simulink model "mrac_model"  (R2022a)
settings: Solver=VariableStepAuto  StartTime=0.0  StopTime=100  RelTol=1e-3
values from neighbouring files (symbols this model uses):
  params = getParamsMRAC(0.5, 1, 10e-8, 0.1, 1)    [mrac.m]
libraries: slctrlblks x1
settings Model: Creator=mateusz  LastModifiedBy=mateusz

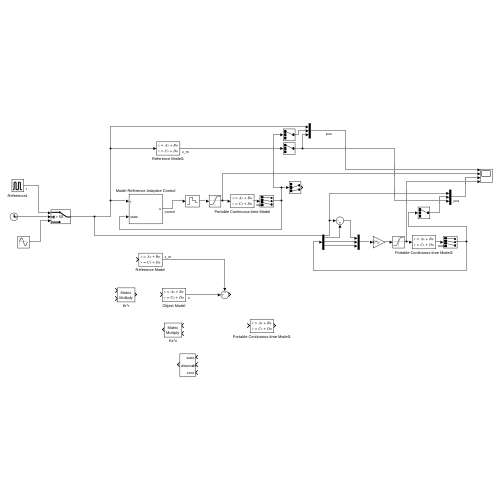
[thumbnail: Simulink's stored preview of the top-level diagram]
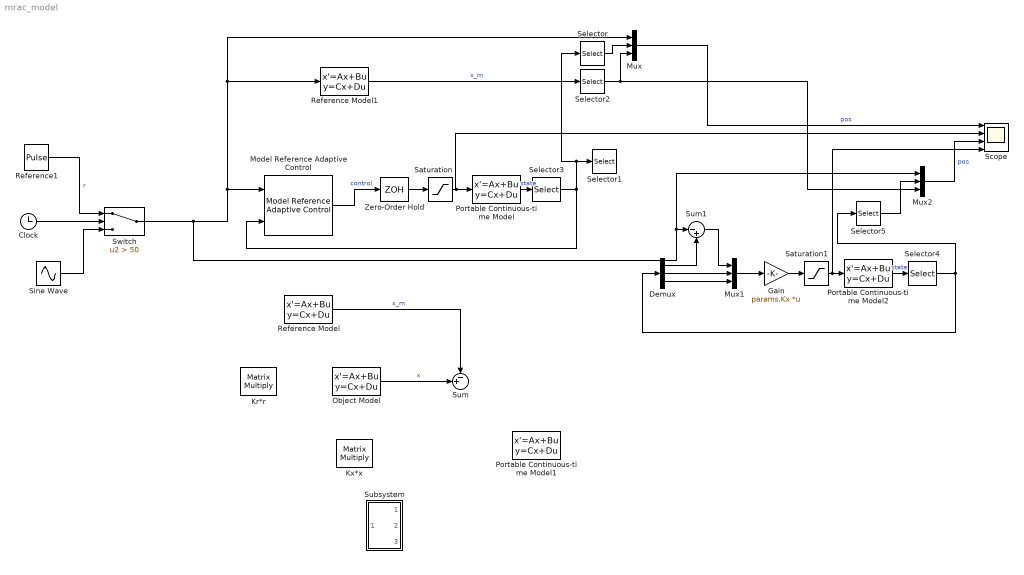
== system mrac_model ==
  Clock : Clock
  Demux : Demux  Outputs=3
  Gain : Gain  Gain=params.Kx  Multiplication=Matrix(K*u)
  Kr*r : Product  Multiplication=Matrix(*)
  Kx*x : Product  Multiplication=Matrix(*)
  Model Reference Adaptive Control : slctrlblks/Model Reference Adaptive Control  selectType=Direct  A=params.A  B=params.B  Ahat=0  ALrEnable=on  gamma_a=1  ALrEnableMod=on  Bhat=1  BLrEnable=on  gamma_b=1  BLrEnableMod=on  externalKtauEnable=off  k_tau=-1  estParamOutput=off  Am=params.A + params.B*params.Kx  Bm=params.B*params.Kr  kx=params.Kx  FBLrEnable=on  gamma_kx=params.gamma_x  FBLrEnableMod=on  kr=params.Kr  FFLrEnable=off  gamma_kr=params.gamma_x  FFLrEnableMod=off  AdaptEnable=on  gamma=params.gamma_w  WLrEnableMod=on  Q=params.Q(1,1)  FeatureTypeOptions=Radial Basis Function  nCen=4  cSpanMin=-1  cSpanMax=1  cSig=5  adaptiveCntrlOutport=off  modChoice=None  sigma_val=0.1
      settings: SourceProductBaseCode=SD
  Mux : Mux  Inputs=3
  Mux1 : Mux  Inputs=3
  Mux2 : Mux  Inputs=3
  Object Model : StateSpace  A=|  B=[0;0;0;2.59e4];  C=eye(4,4)  D=zeros(4,1)  InitialCondition=0
      | [0  1  0    0;
      |      0 -5  4.5  0;
      |      0  0 -0.7108*2  2*23.6012;
      |      0  0 -5.3898 -4040];
  Portable Continuous-time Model : StateSpace  A=|  B=[0;0;0;2.59e4];  C=eye(4,4)  D=zeros(4,1)  InitialCondition=0
      | [0  1  0    0;
      |      0 -5  4.5  0;
      |      0  0 -0.7108*2  2*23.6012;
      |      0  0 -5.3898 -4040];
  Portable Continuous-time Model1 : StateSpace  A=|  B=[0;0;0;2.59e4];  C=eye(4,4)  D=zeros(4,1)  InitialCondition=0
      | [0  1  0    0;
      |      0 -5  4.5  0;
      |      0  0 -0.7108*2  2*23.6012;
      |      0  0 -5.3898 -4040];
  Portable Continuous-time Model2 : StateSpace  A=|  B=[0;0;0;2.59e4];  C=eye(4,4)  D=zeros(4,1)  InitialCondition=0
      | [0  1  0    0;
      |      0 -5  4.5  0;
      |      0  0 -0.7108*2  2*23.6012;
      |      0  0 -5.3898 -4040];
  Reference Model : StateSpace  InitialCondition=0
  Reference Model1 : StateSpace  A=params.Am  B=params.Bm  C=eye(3)  D=zeros(3,1)  InitialCondition=0
  Reference1 : DiscretePulseGenerator  PulseType=Time based  Amplitude=6.28*25  Period=50  PulseWidth=50
  Saturation : Saturate  UpperLimit=1  LowerLimit=-1
  Saturation1 : Saturate  UpperLimit=1  LowerLimit=-1
  Scope : Scope  NumInputPorts=4
  Selector : Selector  InputPortWidth=3  IndexOptions=Index vector (dialog)  Indices=[1]  OutputSizes=1
  Selector1 : Selector  InputPortWidth=3  IndexOptions=Index vector (dialog)  Indices=[2 3]  OutputSizes=1
  Selector2 : Selector  InputPortWidth=3  IndexOptions=Index vector (dialog)  Indices=[1]  OutputSizes=1
  Selector3 : Selector  InputPortWidth=4  IndexOptions=Index vector (dialog)  Indices=[1 2 3]  OutputSizes=1
  Selector4 : Selector  InputPortWidth=4  IndexOptions=Index vector (dialog)  Indices=[1 2 3]  OutputSizes=1
  Selector5 : Selector  InputPortWidth=3  IndexOptions=Index vector (dialog)  Indices=[1]  OutputSizes=1
  Sine Wave : Sin  Amplitude=6.28*25  SampleTime=0
  Subsystem : Subsystem
  Sum : Sum  Inputs=-+|
  Sum1 : Sum  Inputs=|-+
  Switch : Switch  Criteria=u2 > Threshold  Threshold=50  SaturateOnIntegerOverflow=off  InputSameDT=off
  Zero-Order Hold : ZeroOrderHold  SampleTime=0.01
  wires:
  Selector/1 -> Mux/2
  Mux/1 -> Scope/1  "pos"
  Reference Model/1 -> Sum/1  "x_m"
  Object Model/1 -> Sum/2  "x"
  Reference Model1/1 -> Selector2/1  "x_m"
  Selector2/1 -> Mux2/3, Mux/3
  Selector3/1 -> Model Reference Adaptive Control/2, Selector1/1, Selector/1
  Portable Continuous-time Model/1 -> Selector3/1  "state"
  Portable Continuous-time Model2/1 -> Selector4/1  "state"
  Saturation1/1 -> Scope/4, Portable Continuous-time Model2/1
  Gain/1 -> Saturation1/1
  Sum1/1 -> Mux1/1
  Demux/1 -> Sum1/2
  Demux/2 -> Mux1/2
  Demux/3 -> Mux1/3
  Mux1/1 -> Gain/1
  Selector4/1 -> Selector5/1, Demux/1
  Selector5/1 -> Mux2/2
  Mux2/1 -> Scope/3  "pos"
  Switch/1 -> Mux2/1, Sum1/1, Mux/1, Reference Model1/1, Model Reference Adaptive Control/1
  Saturation/1 -> Scope/2, Portable Continuous-time Model/1
  Zero-Order Hold/1 -> Saturation/1
  Model Reference Adaptive Control/1 -> Zero-Order Hold/1  "control"
  Clock/1 -> Switch/2
  Sine Wave/1 -> Switch/3
  Reference1/1 -> Switch/1  "r"

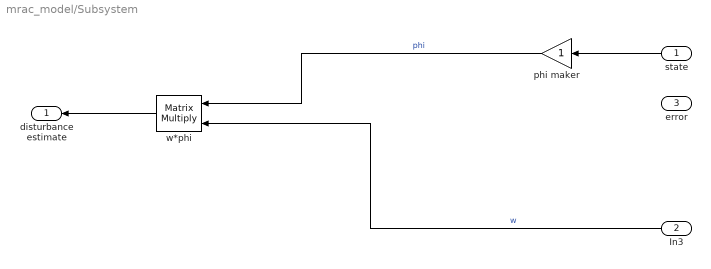
== system mrac_model/Subsystem ==
  state : Inport
  In3 : Inport  Port=2
  error : Inport  Port=3
  phi maker : Gain
  w*phi : Product  Multiplication=Matrix(*)
  disturbance estimate : Outport
  wires:
  w*phi/1 -> disturbance estimate/1
  In3/1 -> w*phi/2  "w"
  state/1 -> phi maker/1
  phi maker/1 -> w*phi/1  "phi"
